simulink model "Template"  (Simulink 7.3)
settings: Solver=ode45  StartTime=0.0  StopTime=10.0  RelTol=1e-3
undefined symbols (not defined in the file): eta1_0_real, v1_0_real, velocitySatValues1
libraries: dspmtrx3 x21, simulink x14, dspindex x5, marine_gnc x4, simulink_extras x1, dspinverses x1
(part 1 of 4)
settings Model: Creator=mcl  LastModifiedBy=mcl

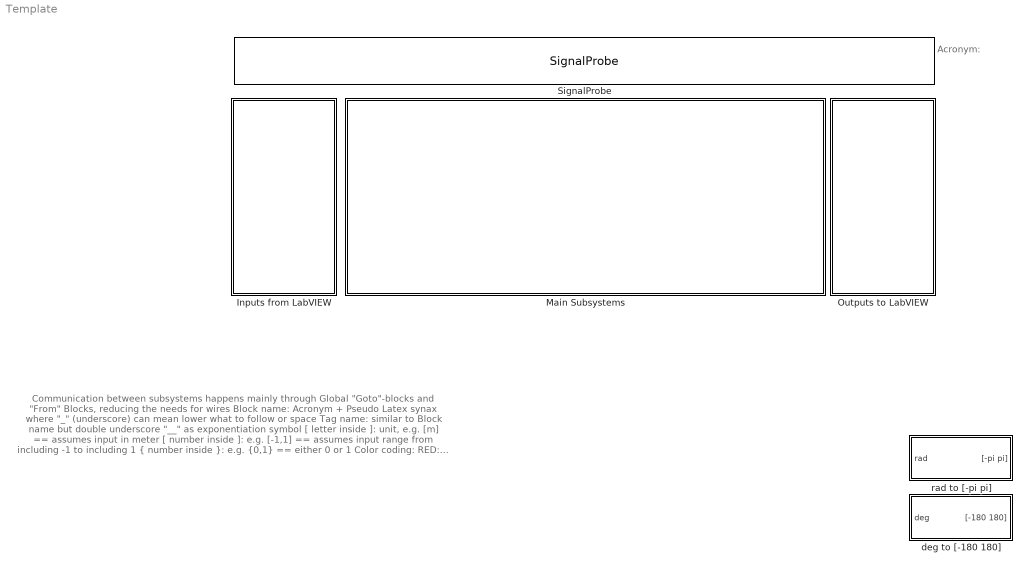
== system Template ==
  note: Communication between subsystems happens mainly through Global "Goto"-blocks and "From" Blocks,
      | reducing the needs for wires
      |
      | Block name: Acronym + Pseudo Latex synax where "_" (underscore) can mean lower what to follow or space
      | Tag name: similar to Block name but double underscore "__" as exponentiation symbol
      |
      | [ letter inside ]: unit, e.g. [m] == assumes input in meter
      | [ number inside ]: e.g. [-1,1] == assumes input range from including -1 to including 1
      | { number inside }:  e.g. {0,1} == either 0 or 1
      |
      | Color coding:
      | RED: Sinks (output ports, terminators, to workspace blocks, etc.)
      | GREEN Sources (inputs ports, constants, etc.)
      | CYAN: Memory blocks: Integrators, unit delays, memory, transfer functions, state space blocks, etc
      | GRAY: Logics blocks: Logic action ports, subsystem enable, etc.
      | ORANGE: GOTO blocks
      | MAGENTA: FROM blocks
      | YELLOW: All remaining blocks,
  note: Acronym:
  Inputs from LabVIEW : Subsystem
  Main Subsystems : Subsystem
  Outputs to LabVIEW : Subsystem
  SignalProbe : S-Function  Description=Use this block with SIT.  FunctionName=SignalProbe  Parameters=1  EnableBusSupport=off
      settings: PreSaveFcn=NISIT_ModelVars;
      mask Description: The LabVIEW Simulation Interface Toolkit uses the SignalProbe block to probe the signals in the model. The SignalProbe block must be on the top level of the model hierarchy. You can have only one SignalProbe block per model file. Do not rename the SignalProbe block. Do not change the name of another model block to SignalProbe.
  deg to [-180 180] : Subsystem
      mask Type: deg to -180/180
      mask Description: Converts an angle in deg to between -180 and 180
      mask Display: disp('[0 360] to [-180 180]')
  rad to [-pi pi] : Subsystem
      mask Type: rad to pi/pi
      mask Description: Converts an angle in rad to between -pi and pi
      mask Display: disp('[0 2pi] to [-pi pi]')

== system Template/Inputs from LabVIEW ==
  Control Input Selector : Constant  Value=0
  Control Mode Selector : Constant  Value=0
  Dynamic Positioning : Subsystem
  Enable CSE1 : Constant  Value=0
  LOS LgV backstepping II : Subsystem
  Linear Simulator : Subsystem
  Path : Subsystem
  PlayStation3 : Subsystem
  tag scope: Control_Input_Selector=global, Control_Mode_Selector=global, Enable_CSE1=global
  wires:
  Control Mode Selector/1 -> [Control_Mode_Selector]
  Control Input Selector/1 -> [Control_Input_Selector]
  Enable CSE1/1 -> [Enable_CSE1]

== system Template/Main Subsystems ==
  C/S Enterprise 1 : Subsystem
  Control : Subsystem
  Guidance : Subsystem
  Naviagation : Subsystem
  Plant : Subsystem

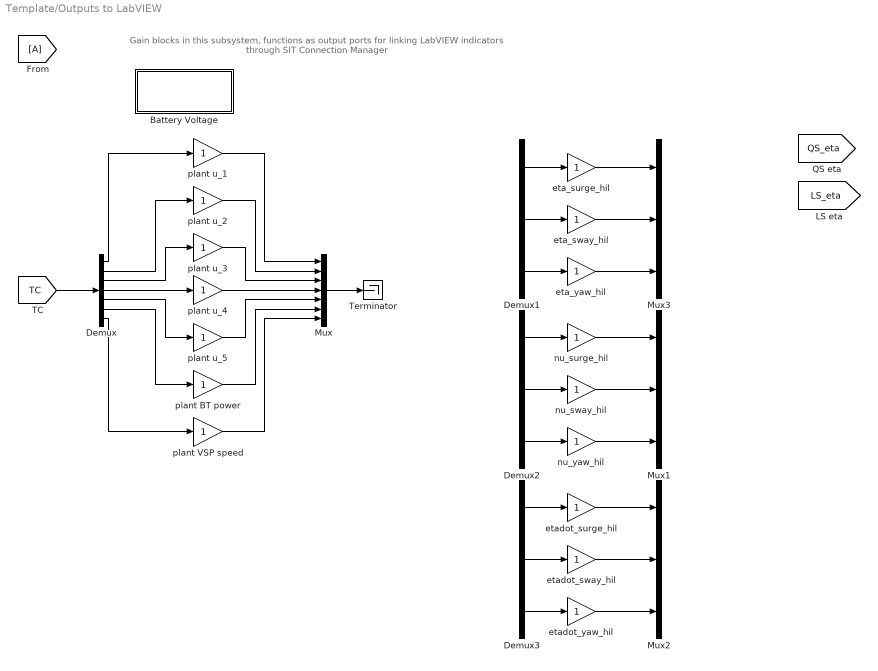
== system Template/Outputs to LabVIEW ==
  note: Gain blocks in this subsystem, functions as output ports for linking LabVIEW indicators through SIT Connection Manager
  Battery Voltage : Subsystem
  Demux : Demux  Outputs=7
  Demux1 : Demux  Outputs=3
  Demux2 : Demux  Outputs=3
  Demux3 : Demux  Outputs=3
  Mux : Mux  Inputs=7
  Mux1 : Mux  Inputs=3
  Mux2 : Mux  Inputs=3
  Mux3 : Mux  Inputs=3
  Terminator : Terminator
  eta_surge_hil : Gain  ParameterDataType=fixdt(1, 16)  ParameterScaling=2^0  OutDataType=fixdt(1, 16)  OutScaling=2^0
  eta_sway_hil : Gain  ParameterDataType=fixdt(1, 16)  ParameterScaling=2^0  OutDataType=fixdt(1, 16)  OutScaling=2^0
  eta_yaw_hil : Gain  ParameterDataType=fixdt(1, 16)  ParameterScaling=2^0  OutDataType=fixdt(1, 16)  OutScaling=2^0
  etadot_surge_hil : Gain  ParameterDataType=fixdt(1, 16)  ParameterScaling=2^0  OutDataType=fixdt(1, 16)  OutScaling=2^0
  etadot_sway_hil : Gain  ParameterDataType=fixdt(1, 16)  ParameterScaling=2^0  OutDataType=fixdt(1, 16)  OutScaling=2^0
  etadot_yaw_hil : Gain  ParameterDataType=fixdt(1, 16)  ParameterScaling=2^0  OutDataType=fixdt(1, 16)  OutScaling=2^0
  nu_surge_hil : Gain  ParameterDataType=fixdt(1, 16)  ParameterScaling=2^0  OutDataType=fixdt(1, 16)  OutScaling=2^0
  nu_sway_hil : Gain  ParameterDataType=fixdt(1, 16)  ParameterScaling=2^0  OutDataType=fixdt(1, 16)  OutScaling=2^0
  nu_yaw_hil : Gain  ParameterDataType=fixdt(1, 16)  ParameterScaling=2^0  OutDataType=fixdt(1, 16)  OutScaling=2^0
  plant BT power : Gain  ParameterDataType=fixdt(1, 16)  ParameterScaling=2^0  OutDataType=fixdt(1, 16)  OutScaling=2^0
  plant VSP speed : Gain  ParameterDataType=fixdt(1, 16)  ParameterScaling=2^0  OutDataType=fixdt(1, 16)  OutScaling=2^0
  plant u_{1..5} (5 alike) : Gain  ParameterDataType=fixdt(1, 16)  ParameterScaling=2^0  OutDataType=fixdt(1, 16)  OutScaling=2^0
  wires:
  Demux/1 -> plant u_1/1
  Demux/2 -> plant u_2/1
  Demux/3 -> plant u_3/1
  Demux/4 -> plant u_4/1
  plant u_4/1 -> Mux/4
  plant u_1/1 -> Mux/1
  plant u_2/1 -> Mux/2
  plant u_3/1 -> Mux/3
  Demux/5 -> plant u_5/1
  Demux/6 -> plant BT power/1
  Demux/7 -> plant VSP speed/1
  plant u_5/1 -> Mux/5
  plant BT power/1 -> Mux/6
  plant VSP speed/1 -> Mux/7
  nu_yaw_hil/1 -> Mux1/3
  nu_sway_hil/1 -> Mux1/2
  nu_surge_hil/1 -> Mux1/1
  Demux2/3 -> nu_yaw_hil/1
  Demux2/2 -> nu_sway_hil/1
  Demux2/1 -> nu_surge_hil/1
  eta_sway_hil/1 -> Mux3/2
  eta_yaw_hil/1 -> Mux3/3
  eta_surge_hil/1 -> Mux3/1
  Demux1/3 -> eta_yaw_hil/1
  Demux1/2 -> eta_sway_hil/1
  Demux1/1 -> eta_surge_hil/1
  etadot_sway_hil/1 -> Mux2/2
  etadot_yaw_hil/1 -> Mux2/3
  etadot_surge_hil/1 -> Mux2/1
  Demux3/3 -> etadot_yaw_hil/1
  Demux3/2 -> etadot_sway_hil/1
  Demux3/1 -> etadot_surge_hil/1
  [TC] -> Demux/1
  Mux/1 -> Terminator/1

== system Template/deg to [-180 180] ==
  deg : Inport  OutDataType=sfix(16)  OutScaling=2^0
  Constant : Constant  Value=2*180  OutDataType=sfix(16)  OutScaling=2^0
  Gain : Gain  Gain=180  ParameterDataType=sfix(16)  ParameterScaling=2^0  OutDataType=sfix(16)  OutScaling=2^0  SaturateOnIntegerOverflow=on  OutDataTypeStr=Inherit: Same as input  ParamDataTypeStr=Inherit: Same as input
  Math Function : Math  Operator=rem  OutDataType=sfix(16)  OutScaling=2^0  SaturateOnIntegerOverflow=on
  Saturation : Saturate  UpperLimit=1e10  LowerLimit=-1e10
  Sign : Signum
  Sum : Sum  Inputs=|+-  OutDataType=sfix(16)  OutScaling=2^0  SaturateOnIntegerOverflow=on
  Sum1 : Sum  Inputs=|++  OutDataType=sfix(16)  OutScaling=2^0  SaturateOnIntegerOverflow=on
  "[-180 180]" : Outport  OutDataType=sfix(16)  OutScaling=2^0
  wires:
  Sum/1 -> "[-180 180]"/1
  Math Function/1 -> Sum/1
  Constant/1 -> Math Function/2
  Sum1/1 -> Math Function/1
  Gain/1 -> Sum1/2, Sum/2
  Sign/1 -> Gain/1
  deg/1 -> Saturation/1
  Saturation/1 -> Sign/1, Sum1/1

== system Template/rad to [-pi pi] ==
  rad : Inport  OutDataType=sfix(16)  OutScaling=2^0
  Constant : Constant  Value=2*pi  OutDataType=sfix(16)  OutScaling=2^0
  Gain : Gain  Gain=pi  ParameterDataType=sfix(16)  ParameterScaling=2^0  OutDataType=sfix(16)  OutScaling=2^0  SaturateOnIntegerOverflow=on  OutDataTypeStr=Inherit: Same as input  ParamDataTypeStr=Inherit: Same as input
  Math Function : Math  Operator=rem  OutDataType=sfix(16)  OutScaling=2^0  SaturateOnIntegerOverflow=on
  Saturation : Saturate  UpperLimit=1e10  LowerLimit=-1e10
  Sign : Signum
  Sum : Sum  Inputs=|+-  OutDataType=sfix(16)  OutScaling=2^0  SaturateOnIntegerOverflow=on
  Sum1 : Sum  Inputs=|++  OutDataType=sfix(16)  OutScaling=2^0  SaturateOnIntegerOverflow=on
  "[-pi pi]" : Outport  OutDataType=sfix(16)  OutScaling=2^0
  wires:
  Saturation/1 -> Sum1/1, Sign/1
  rad/1 -> Saturation/1
  Sign/1 -> Gain/1
  Gain/1 -> Sum/2, Sum1/2
  Sum1/1 -> Math Function/1
  Constant/1 -> Math Function/2
  Math Function/1 -> Sum/1
  Sum/1 -> "[-pi pi]"/1

== system Template/Inputs from LabVIEW/Dynamic Positioning ==
  K_d : Subsystem
  K_d_Surge : Constant  Value=50
  K_d_Sway : Constant  Value=30
  K_d_Yaw : Constant  Value=5
  K_i : Subsystem
  K_i_Surge : Constant  Value=0
  K_i_Sway : Constant  Value=0
  K_i_Yaw : Constant  Value=0
  K_p : Subsystem
  K_p_Surge : Constant  Value=2*1.5*2
  K_p_Sway : Constant  Value=2*10*2
  K_p_Yaw : Constant  Value=0.5*3
  Reset integrator : Constant  Value=0
  Setpoint : Subsystem
  tag scope: DP_Reset_integrator=global
  wires:
  Reset integrator/1 -> [DP_Reset_integrator]
  K_p_Surge/1 -> K_p/1(11)
  K_p_Sway/1 -> K_p/2(22)
  K_p_Yaw/1 -> K_p/3(33)
  K_d_Surge/1 -> K_d/1(11)
  K_d_Sway/1 -> K_d/2(22)
  K_d_Yaw/1 -> K_d/3(33)
  K_i_Surge/1 -> K_i/1(11)
  K_i_Sway/1 -> K_i/2(22)
  K_i_Yaw/1 -> K_i/3(33)

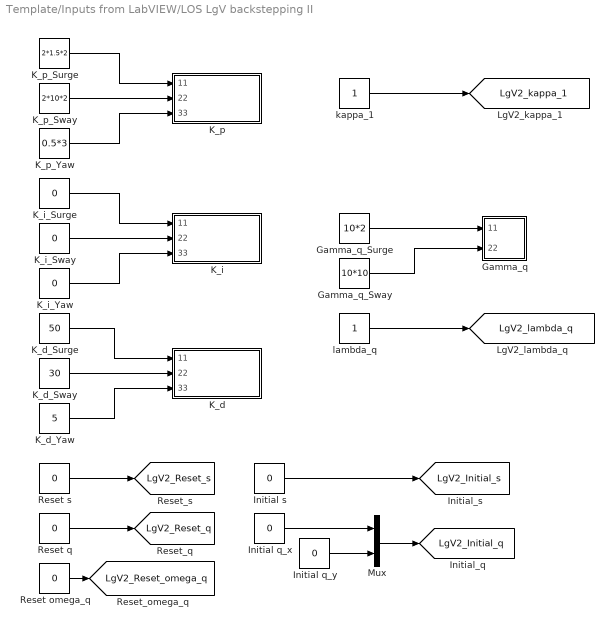
== system Template/Inputs from LabVIEW/LOS LgV backstepping II ==
  Gamma_q : Subsystem
  Gamma_q_Surge : Constant  Value=10*2
  Gamma_q_Sway : Constant  Value=10*10
  Initial q_x : Constant  Value=0  OutDataType=fixdt(1, 16)  OutScaling=2^0
  Initial q_y : Constant  Value=0  OutDataType=fixdt(1, 16)  OutScaling=2^0
  Initial s : Constant  Value=0  OutDataType=fixdt(1, 16)  OutScaling=2^0
  K_d : Subsystem
  K_d_Surge : Constant  Value=50
  K_d_Sway : Constant  Value=30
  K_d_Yaw : Constant  Value=5
  K_i : Subsystem
  K_i_Surge : Constant  Value=0
  K_i_Sway : Constant  Value=0
  K_i_Yaw : Constant  Value=0
  K_p : Subsystem
  K_p_Surge : Constant  Value=2*1.5*2
  K_p_Sway : Constant  Value=2*10*2
  K_p_Yaw : Constant  Value=0.5*3
  Mux : Mux  Inputs=2
  Reset omega_q : Constant  Value=0
  Reset q : Constant  Value=0
  Reset s : Constant  Value=0
  kappa_1 : Constant
  lambda_q : Constant
  tag scope: LgV2_Initial_q=global, LgV2_Initial_s=global, LgV2_Reset_omega_q=global, LgV2_Reset_q=global, LgV2_Reset_s=global, LgV2_kappa_1=global, LgV2_lambda_q=global
  wires:
  K_p_Surge/1 -> K_p/1(11)
  K_p_Sway/1 -> K_p/2(22)
  K_p_Yaw/1 -> K_p/3(33)
  K_d_Surge/1 -> K_d/1(11)
  K_d_Sway/1 -> K_d/2(22)
  K_d_Yaw/1 -> K_d/3(33)
  K_i_Surge/1 -> K_i/1(11)
  K_i_Sway/1 -> K_i/2(22)
  K_i_Yaw/1 -> K_i/3(33)
  Gamma_q_Surge/1 -> Gamma_q/1(11)
  Gamma_q_Sway/1 -> Gamma_q/2(22)
  kappa_1/1 -> [LgV2_kappa_1]
  lambda_q/1 -> [LgV2_lambda_q]
  Initial q_x/1 -> Mux/1
  Initial q_y/1 -> Mux/2
  Reset s/1 -> [LgV2_Reset_s]
  Reset q/1 -> [LgV2_Reset_q]
  Initial s/1 -> [LgV2_Initial_s]
  Mux/1 -> [LgV2_Initial_q]
  Reset omega_q/1 -> [LgV2_Reset_omega_q]

== system Template/Inputs from LabVIEW/Linear Simulator ==
  note: Enable Linear Simulator: Activation
      | Reset Linear Simulator integrator: Reset
      | Initial u: Initial speed in surge
      | Initial v: Initial speed in sway
      | Initial r: Initial speed in yaw
      | Initial x: Initial position in surge
      | Initial y: Initial position in sway
      | Initial psi: Initial heading
  Enable Linear Simulator : Constant  Value=0
  Initial psi [rad] : Constant  Value=0  OutDataType=fixdt(1, 16)  OutScaling=2^0
  Initial r [rad/s] : Constant  Value=0  OutDataType=fixdt(1, 16)  OutScaling=2^0
  Initial u [m/s] : Constant  Value=0  OutDataType=fixdt(1, 16)  OutScaling=2^0
  Initial v [m/s] : Constant  Value=0  OutDataType=fixdt(1, 16)  OutScaling=2^0
  Initial x [m] : Constant  Value=0  OutDataType=fixdt(1, 16)  OutScaling=2^0
  Initial y [m] : Constant  Value=0  OutDataType=fixdt(1, 16)  OutScaling=2^0
  Mux : Mux  Inputs=3
  Mux1 : Mux  Inputs=3
  Reset Linear Simulator integrator : Constant  Value=0
  tag scope: LS_Enable=global, LS_Initial_eta=global, LS_Initial_nu=global, LS_Reset=global
  wires:
  Enable Linear Simulator/1 -> [LS_Enable]
  Reset Linear Simulator integrator/1 -> [LS_Reset]
  Mux/1 -> [LS_Initial_nu]
  Initial r [rad/s]/1 -> Mux/3
  Initial v [m/s]/1 -> Mux/2
  Initial u [m/s]/1 -> Mux/1
  Mux1/1 -> [LS_Initial_eta]
  Initial psi [rad]/1 -> Mux1/3
  Initial y [m]/1 -> Mux1/2
  Initial x [m]/1 -> Mux1/1

== system Template/Inputs from LabVIEW/Path ==
  note: u_d: Desired surge speed of vessel
      | Path Selector: Workaround parameter for switching between linear path(==0) and ellipse path(==1)
      | x_dmax: Upper limit of desired x-ooordinate
      | x_dmin: Lower limit of desired x-coordiante
      | y_dmax: Upper limit of desired y-ooordinate
      | y_dmin: Lower limit of desired y-coordiante
      | Delta: Lookahead distance for LOS guidance
      | my: Gradient path minimizing tuning value
  Delta [m] : Constant  Value=2  OutDataType=fixdt(1, 16)  OutScaling=2^0
  Ellipse : Subsystem
  Linear : Subsystem
  Path Selector  [-] : Constant  Value=0
  my [-] : Constant  Value=10  OutDataType=fixdt(1, 16)  OutScaling=2^0
  u_d [m] : Constant  Value=0.15  OutDataType=fixdt(1, 16)  OutScaling=2^0
  x_dmax [m] : Constant  Value=40
  x_dmin [m] : Constant  Value=-40
  y_dmax [m] : Constant  Value=7
  y_dmin [m] : Constant  Value=-7
  tag scope: Delta=global, Path_Selector=global, my=global, u_d=global, x_dmax=global, x_dmin=global, y_dmax=global, y_dmin=global
  wires:
  u_d [m]/1 -> [u_d]  "Desired speed [m/s]"
  Delta [m]/1 -> [Delta]  "Lookahead distance [m]"
  my [-]/1 -> [my]  "s tuning parameter"
  Path Selector  [-]/1 -> [Path_Selector]  "chosen path {0,1}"
  x_dmax [m]/1 -> [x_dmax]
  x_dmin [m]/1 -> [x_dmin]
  y_dmax [m]/1 -> [y_dmax]
  y_dmin [m]/1 -> [y_dmin]

== system Template/Inputs from LabVIEW/PlayStation3 ==
  note: Postive Y-axis of analog sticks points up (in the direction of the shoulder buttons)
      | Postive X-axis of analog sticks points to the right (in the direction of Triange, Circle, X and Square buttons)
      |
      | AS_LX: PS3 Analog Stick Left X-postition
      | AS_LY: PS3 Analog Stick Left Y-postition
      | AS_RX: PS3 Analog Stick Right X-postition
      | AS_RY: PS3 Analog Stick Right Y-postition
      | L2: PS3 bottom left sholderbutton
      | R2: PS3 bottom right shoulderbotton
      | PS3_BT_Power: PS3 command bow thruster power setpoint
      | PS3 _VSP_speed: PS3 command Voith Schneider Propeller speed
  "AS_LX [-] " : Constant  Value=0
  AS_LY [-] : Constant  Value=0
  AS_RX [-] : Constant  Value=0
  AS_RY [-] : Constant  Value=0
  L2 [-] : Constant  Value=0
  PS3_BT_Power  [-] : Constant  Value=0
  PS3_VSP_Speed  [-] : Constant  Value=0
  R2 [-] : Constant  Value=0
  ScalingLX : Gain  Gain=1/32767
  ScalingLY : Gain  Gain=1/32767
  ScalingRY : Gain  Gain=1/32767
  Scaling_RX : Gain  Gain=1/32767
  tag scope: PS3_AS_LX=global, PS3_AS_LY=global, PS3_AS_RX=global, PS3_AS_RY=global, PS3_BT_Power=global, PS3_L2=global, PS3_R2=global, PS3_VSP_Speed=global
  wires:
  PS3_VSP_Speed  [-]/1 -> [PS3_VSP_Speed]  "Voith Schnider Propeller Speed"
  PS3_BT_Power  [-]/1 -> [PS3_BT_Power]  "Bow Thruster Power"
  "AS_LX [-] "/1 -> ScalingLX/1  "x-position of left analog stick [-32767,32767]"
  ScalingLX/1 -> [PS3_AS_LX]  "x-position of left analog stick [-1,1]"
  AS_LY [-]/1 -> ScalingLY/1  "y-position of left analog stick [-32767,32767]"
  ScalingLY/1 -> [PS3_AS_LY]  "y-position of left analog stick [-1,1]"
  AS_RX [-]/1 -> Scaling_RX/1  "x-position of right analog stick  [-32767,32767]"
  Scaling_RX/1 -> [PS3_AS_RX]  "x-position of right analog stick  [-1,1]"
  ScalingRY/1 -> [PS3_AS_RY]  "y-position of right analog stick [-1,1]"
  AS_RY [-]/1 -> ScalingRY/1  "y-position of right analog stick [-32767,32767]"
  L2 [-]/1 -> [PS3_L2]  "L2 Button [-1,0]"
  R2 [-]/1 -> [PS3_R2]  "R2 Button [0,1]"

== system Template/Main Subsystems/C/S Enterprise 1 ==
  Linear dampning matrix : Subsystem
  Mass matrix : Subsystem
  Thruster configuration matrix : Subsystem
  tag scope: B=global, D_L=global, M=global
  wires:
  Mass matrix/1(M) -> [M]
  Linear dampning matrix/1(D_L) -> [D_L]
  Thruster configuration matrix/1(B) -> [B]

== system Template/Main Subsystems/Control ==
  Control Switch : Subsystem
  DP control : Subsystem
  LgV2 : Subsystem
  Thruster allocation : Subsystem

== system Template/Main Subsystems/Guidance ==
  Line-Of-Sight Path-Following : Subsystem

== system Template/Main Subsystems/Naviagation ==
  Input from SIT : Subsystem
  Navigation Switch : Subsystem

== system Template/Main Subsystems/Plant ==
  CSE1 : Subsystem
  Enable CSE1 : Constant  Value=0
  Enable Linear Simulator : Constant  Value=0
  Inverse : Product  Inputs=/  Multiplication=Matrix(*)
  Linear Simulator : Subsystem
      settings: MinAlgLoopOccurrences=on
  saturation : Subsystem
  tag scope: LS_eta=global, LS_etadot=global, LS_nu=global
  wires:
  Enable CSE1/1 -> CSE1/Enable
  Enable Linear Simulator/1 -> Linear Simulator/Enable
  saturation/1(sat_tau) -> Linear Simulator/1(tau)
  [tau] -> saturation/1(tau)
  [TC] -> CSE1/1(Thurster setting)
  Linear Simulator/1(eta_hil) -> [LS_eta]
  Linear Simulator/2(nu_hil) -> [LS_nu]
  Linear Simulator/3(etadot_hil) -> [LS_etadot]
  [M] -> Inverse/1
  Inverse/1 -> Linear Simulator/2(M_inv)
  [D_L] -> Linear Simulator/3(D_L)
  [LS_Reset] -> Linear Simulator/4(Reset)
  [LS_Initial_eta] -> Linear Simulator/5(eta_0)
  [LS_Initial_nu] -> Linear Simulator/6(nu_0)

== system Template/Outputs to LabVIEW/Battery Voltage ==
  note: Main battery is multipled by 2, since the voltage is halfed at measuring point
  Battery Bow Thruster : Gain  ParameterDataType=fixdt(1, 16)  ParameterScaling=2^0  OutDataType=fixdt(1, 16)  OutScaling=2^0
  Battery Main : Gain  Gain=2  ParameterDataType=fixdt(1, 16)  ParameterScaling=2^0  OutDataType=fixdt(1, 16)  OutScaling=2^0
  Battery Servo : Gain  ParameterDataType=fixdt(1, 16)  ParameterScaling=2^0  OutDataType=fixdt(1, 16)  OutScaling=2^0
  Terminator Bow Thruster Battery : Terminator
  Terminator Main Battery : Terminator
  Terminator Servo Battery : Terminator
  wires:
  [Battery_BT] -> Battery Bow Thruster/1
  Battery Bow Thruster/1 -> Terminator Bow Thruster Battery/1
  [Battery_Servo] -> Battery Servo/1
  Battery Servo/1 -> Terminator Servo Battery/1
  [Battery_Main] -> Battery Main/1
  Battery Main/1 -> Terminator Main Battery/1

== system Template/Inputs from LabVIEW/Dynamic Positioning/K_d ==
  note: Creating 3x3 diagonal matrix
  11 : Inport
  22 : Inport  Port=2
  33 : Inport  Port=3
  {12..13,21,23,31..32} (6 alike) : Constant  Value=0
  Mux : Mux  Inputs=9
  "[3x3]" : Reshape  OutputDimensionality=Customize  OutputDimensions=[3,3]
  tag scope: DP_K_d=global
  wires:
  "[3x3]"/1 -> [DP_K_d]
  33/1 -> Mux/9
  23/1 -> Mux/8
  13/1 -> Mux/7
  32/1 -> Mux/6
  22/1 -> Mux/5
  12/1 -> Mux/4
  31/1 -> Mux/3
  21/1 -> Mux/2
  11/1 -> Mux/1
  Mux/1 -> "[3x3]"/1

== system Template/Inputs from LabVIEW/Dynamic Positioning/K_i ==
  note: Creating 3x3 diagonal matrix
  11 : Inport
  22 : Inport  Port=2
  33 : Inport  Port=3
  {12..13,21,23,31..32} (6 alike) : Constant  Value=0
  Mux : Mux  Inputs=9
  "[3x3]" : Reshape  OutputDimensionality=Customize  OutputDimensions=[3,3]
  tag scope: DP_K_i=global
  wires:
  "[3x3]"/1 -> [DP_K_i]
  33/1 -> Mux/9
  23/1 -> Mux/8
  13/1 -> Mux/7
  32/1 -> Mux/6
  22/1 -> Mux/5
  12/1 -> Mux/4
  31/1 -> Mux/3
  21/1 -> Mux/2
  11/1 -> Mux/1
  Mux/1 -> "[3x3]"/1

== system Template/Inputs from LabVIEW/Dynamic Positioning/K_p ==
  note: Creating 3x3 diagonal matrix
  11 : Inport
  22 : Inport  Port=2
  33 : Inport  Port=3
  {12..13,21,23,31..32} (6 alike) : Constant  Value=0
  Mux : Mux  Inputs=9
  "[3x3]" : Reshape  OutputDimensionality=Customize  OutputDimensions=[3,3]
  tag scope: DP_K_p=global
  wires:
  Mux/1 -> "[3x3]"/1
  11/1 -> Mux/1
  21/1 -> Mux/2
  31/1 -> Mux/3
  12/1 -> Mux/4
  22/1 -> Mux/5
  32/1 -> Mux/6
  13/1 -> Mux/7
  23/1 -> Mux/8
  33/1 -> Mux/9
  "[3x3]"/1 -> [DP_K_p]

== system Template/Inputs from LabVIEW/Dynamic Positioning/Setpoint ==
  " y_d [m]" : Constant  Value=0
  Degrees to Radians : simulink_extras/Transformations/Degrees to Radians  SystemSampleTime=-1
  Mux : Mux  Inputs=3
  psi_d [deg] : Constant  Value=0
  x_d [m] : Constant  Value=0
  tag scope: Setpoint=global
  wires:
  Degrees to Radians/1 -> Mux/3
  psi_d [deg]/1 -> Degrees to Radians/1
  " y_d [m]"/1 -> Mux/2
  x_d [m]/1 -> Mux/1
  Mux/1 -> [Setpoint]

== system Template/Inputs from LabVIEW/LOS LgV backstepping II/Gamma_q ==
  11 : Inport
  22 : Inport  Port=2
  12 : Constant  Value=0
  21 : Constant  Value=0
  Mux : Mux
  "[2x2]" : Reshape  OutputDimensionality=Customize  OutputDimensions=[2,2]
  tag scope: LgV2_Gamma_q=global
  wires:
  Mux/1 -> "[2x2]"/1
  11/1 -> Mux/1
  21/1 -> Mux/2
  12/1 -> Mux/3
  22/1 -> Mux/4
  "[2x2]"/1 -> [LgV2_Gamma_q]

== system Template/Inputs from LabVIEW/LOS LgV backstepping II/K_d ==
  note: Creating 3x3 diagonal matrix
  11 : Inport
  22 : Inport  Port=2
  33 : Inport  Port=3
  {12..13,21,23,31..32} (6 alike) : Constant  Value=0
  Mux : Mux  Inputs=9
  "[3x3]" : Reshape  OutputDimensionality=Customize  OutputDimensions=[3,3]
  tag scope: LgV2_K_d=global
  wires:
  "[3x3]"/1 -> [LgV2_K_d]
  33/1 -> Mux/9
  23/1 -> Mux/8
  13/1 -> Mux/7
  32/1 -> Mux/6
  22/1 -> Mux/5
  12/1 -> Mux/4
  31/1 -> Mux/3
  21/1 -> Mux/2
  11/1 -> Mux/1
  Mux/1 -> "[3x3]"/1

== system Template/Inputs from LabVIEW/LOS LgV backstepping II/K_i ==
  note: Creating 3x3 diagonal matrix
  11 : Inport
  22 : Inport  Port=2
  33 : Inport  Port=3
  {12..13,21,23,31..32} (6 alike) : Constant  Value=0
  Mux : Mux  Inputs=9
  "[3x3]" : Reshape  OutputDimensionality=Customize  OutputDimensions=[3,3]
  tag scope: LgV2_K_i=global
  wires:
  "[3x3]"/1 -> [LgV2_K_i]
  33/1 -> Mux/9
  23/1 -> Mux/8
  13/1 -> Mux/7
  32/1 -> Mux/6
  22/1 -> Mux/5
  12/1 -> Mux/4
  31/1 -> Mux/3
  21/1 -> Mux/2
  11/1 -> Mux/1
  Mux/1 -> "[3x3]"/1

== system Template/Inputs from LabVIEW/LOS LgV backstepping II/K_p ==
  note: Creating 3x3 diagonal matrix
  11 : Inport
  22 : Inport  Port=2
  33 : Inport  Port=3
  {12..13,21,23,31..32} (6 alike) : Constant  Value=0
  Mux : Mux  Inputs=9
  "[3x3]" : Reshape  OutputDimensionality=Customize  OutputDimensions=[3,3]
  tag scope: LgV2_K_p=global
  wires:
  Mux/1 -> "[3x3]"/1
  11/1 -> Mux/1
  21/1 -> Mux/2
  31/1 -> Mux/3
  12/1 -> Mux/4
  22/1 -> Mux/5
  32/1 -> Mux/6
  13/1 -> Mux/7
  23/1 -> Mux/8
  33/1 -> Mux/9
  "[3x3]"/1 -> [LgV2_K_p]

== system Template/Inputs from LabVIEW/Path/Ellipse ==
  note: origin_x: ellipse origin x-coordinate
      | origin_y: ellipse origin y-coordinate
      | r_x: ellipse radius x-direction
      | r_y: ellipse radius y-direction
      | k: step scaling factor of path parameter
  k [-] : Constant  Value=pi/180*2  OutDataType=fixdt(1, 16)  OutScaling=2^0
  origin_x [m] : Constant  Value=4.5  OutDataType=fixdt(1, 16)  OutScaling=2^0
  origo_y [m] : Constant  Value=0  OutDataType=fixdt(1, 16)  OutScaling=2^0
  r_x [m] : Constant  Value=5.5  OutDataType=fixdt(1, 16)  OutScaling=2^0
  r_y [m] : Constant  Value=2  OutDataType=fixdt(1, 16)  OutScaling=2^0
  tag scope: k=global, origin_x=global, origin_y=global, r_x=global, r_y=global
  wires:
  origin_x [m]/1 -> [origin_x]  "x-coord. origin ellipse path [m]"
  origo_y [m]/1 -> [origin_y]  "y-coord. origin ellipse path [m]"
  r_x [m]/1 -> [r_x]  "radius ellipse path x-axis [m]"
  r_y [m]/1 -> [r_y]  "radius ellipse path y-axis [m]"
  k [-]/1 -> [k]  "step scaling factor ellipse path [-]"

== system Template/Inputs from LabVIEW/Path/Linear ==
  note: x_1: reference way-point x-coordinate
      | y_1: reference way-point y-coordinate
      | x_2: direction way-point x-coordinate
      | y_2: direction way-point y-coordinate
  x_1 [m] : Constant  Value=0  OutDataType=fixdt(1, 16)  OutScaling=2^0
  x_2 [m] : Constant  Value=5.5  OutDataType=fixdt(1, 16)  OutScaling=2^0
  y_1 [m] : Constant  Value=0  OutDataType=fixdt(1, 16)  OutScaling=2^0
  y_2 [m] : Constant  Value=2  OutDataType=fixdt(1, 16)  OutScaling=2^0
  tag scope: x_1=global, x_2=global, y_1=global, y_2=global
  wires:
  x_1 [m]/1 -> [x_1]  "x-coord. reference point path [m]"
  y_1 [m]/1 -> [y_1]  "y-coord, reference point path [m]"
  x_2 [m]/1 -> [x_2]  "x-coord, direction point path [m]"
  y_2 [m]/1 -> [y_2]  "y-coord, direction point path [m]"

== system Template/Main Subsystems/C/S Enterprise 1/Linear dampning matrix ==
  -N_r : Gain  Gain=-1  ParameterDataType=fixdt(1, 16)  ParameterScaling=2^0  OutDataType=fixdt(1, 16)  OutScaling=2^0
  -N_v : Gain  Gain=-1  ParameterDataType=fixdt(1, 16)  ParameterScaling=2^0  OutDataType=fixdt(1, 16)  OutScaling=2^0
  -X_u : Gain  Gain=-1  ParameterDataType=fixdt(1, 16)  ParameterScaling=2^0  OutDataType=fixdt(1, 16)  OutScaling=2^0
  -Y_v : Gain  Gain=-1  ParameterDataType=fixdt(1, 16)  ParameterScaling=2^0  OutDataType=fixdt(1, 16)  OutScaling=2^0
  -Y_vr : Gain  Gain=-1  ParameterDataType=fixdt(1, 16)  ParameterScaling=2^0  OutDataType=fixdt(1, 16)  OutScaling=2^0
  D_L_{12..13,21,31} (4 alike) : Constant  Value=0
  Linear Dampning matrix : Reshape  OutputDimensionality=Customize  OutputDimensions=[3,3]
  Mux : Mux  Inputs=9
  N_r : Constant  Value=-1.900
  N_v : Constant  Value=0.18140
  X_u : Constant  Value=-0.59739
  Y_r : Constant  Value=-7.250
  Y_v : Constant  Value=-3.50625
  D_L : Outport
  wires:
  -N_r/1 -> Mux/9
  -Y_vr/1 -> Mux/8
  D_L_13/1 -> Mux/7
  -N_v/1 -> Mux/6
  -Y_v/1 -> Mux/5
  D_L_12/1 -> Mux/4
  D_L_31/1 -> Mux/3
  D_L_21/1 -> Mux/2
  -X_u/1 -> Mux/1
  N_r/1 -> -N_r/1
  Y_r/1 -> -Y_vr/1
  N_v/1 -> -N_v/1
  Y_v/1 -> -Y_v/1
  Linear Dampning matrix/1 -> D_L/1
  Mux/1 -> Linear Dampning matrix/1
  X_u/1 -> -X_u/1

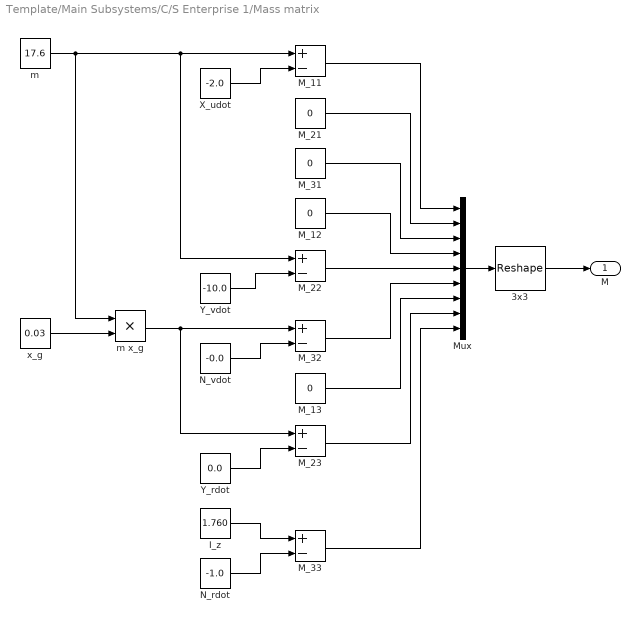
== system Template/Main Subsystems/C/S Enterprise 1/Mass matrix ==
  3x3 : Reshape  OutputDimensionality=Customize  OutputDimensions=[3,3]
  I_z : Constant  Value=1.760
  M_{11,22..23,32..33} (5 alike) : Sum  Inputs=+-
  M_{12..13,21,31} (4 alike) : Constant  Value=0
  Mux : Mux  Inputs=9
  N_rdot : Constant  Value=-1.0
  N_vdot : Constant  Value=-0.0
  X_udot : Constant  Value=-2.0
  Y_rdot : Constant  Value=0.0
  Y_vdot : Constant  Value=-10.0
  m : Constant  Value=17.6
  m x_g : Product  RndMeth=Zero
  x_g : Constant  Value=0.03
  M : Outport
  wires:
  3x3/1 -> M/1
  Mux/1 -> 3x3/1
  M_33/1 -> Mux/9
  M_23/1 -> Mux/8
  M_13/1 -> Mux/7
  M_32/1 -> Mux/6
  M_22/1 -> Mux/5
  M_12/1 -> Mux/4
  M_31/1 -> Mux/3
  M_21/1 -> Mux/2
  M_11/1 -> Mux/1
  N_rdot/1 -> M_33/2
  I_z/1 -> M_33/1
  Y_rdot/1 -> M_23/2
  N_vdot/1 -> M_32/2
  m x_g/1 -> M_23/1, M_32/1
  x_g/1 -> m x_g/2
  Y_vdot/1 -> M_22/2
  X_udot/1 -> M_11/2
  m/1 -> m x_g/1, M_22/1, M_11/1

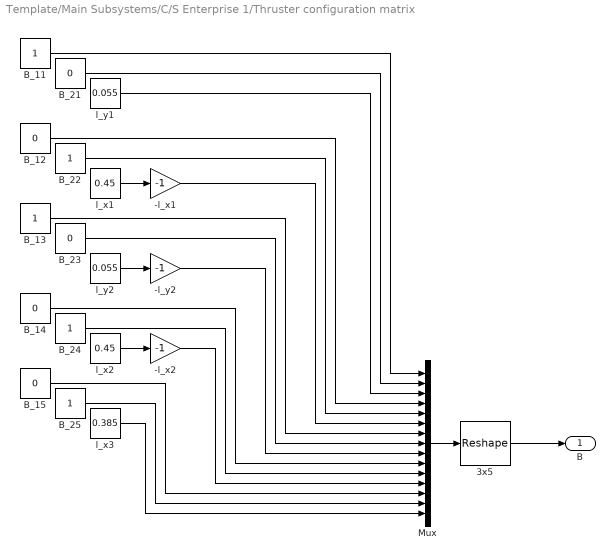
== system Template/Main Subsystems/C/S Enterprise 1/Thruster configuration matrix ==
  -l_x1 : Gain  Gain=-1
  -l_x2 : Gain  Gain=-1
  -l_y2 : Gain  Gain=-1
  3x5 : Reshape  OutputDimensionality=Customize  OutputDimensions=[3,5]
  B_{11,13,22,24..25} (5 alike) : Constant
  B_{12,14..15,21,23} (5 alike) : Constant  Value=0
  Mux : Mux  Inputs=15
  l_x1 : Constant  Value=0.45
  l_x2 : Constant  Value=0.45
  l_x3 : Constant  Value=0.385
  l_y1 : Constant  Value=0.055
  l_y2 : Constant  Value=0.055
  B : Outport
  wires:
  l_x3/1 -> Mux/15
  B_25/1 -> Mux/14
  B_15/1 -> Mux/13
  -l_x2/1 -> Mux/12
  -l_y2/1 -> Mux/9
  -l_x1/1 -> Mux/6
  l_x2/1 -> -l_x2/1
  B_24/1 -> Mux/11
  B_14/1 -> Mux/10
  l_y2/1 -> -l_y2/1
  B_23/1 -> Mux/8
  B_13/1 -> Mux/7
  l_x1/1 -> -l_x1/1
  B_22/1 -> Mux/5
  B_12/1 -> Mux/4
  l_y1/1 -> Mux/3
  B_21/1 -> Mux/2
  B_11/1 -> Mux/1
  3x5/1 -> B/1
  Mux/1 -> 3x5/1

== system Template/Main Subsystems/Control/Control Switch ==
  note: 0 - PS3 u input control
      | 1 - DP control
      | 2 - LgV2 control
  Control Mode : Constant  Value=0
  tau Switch : MultiPortSwitch  Inputs=2  zeroidx=on
  tag scope: tau=global
  wires:
  Control Mode/1 -> tau Switch/1
  [DP_tau] -> tau Switch/2
  [LgV2_tau] -> tau Switch/3
  tau Switch/1 -> [tau]

== system Template/Main Subsystems/Control/DP control ==
  note: Modified version of the DP control found in MSS toolbx
  Demux : Demux  Outputs=3
  Integrator : Integrator  ExternalReset=level
  Mux : Mux  Inputs=3
  Product : Product  Multiplication=Matrix(*)  OutDataType=fixdt(1, 16)  OutScaling=2^0  RndMeth=Zero
  Product1 : Product  Multiplication=Matrix(*)  OutDataType=fixdt(1, 16)  OutScaling=2^0  RndMeth=Zero
  Product2 : Product  Multiplication=Matrix(*)  OutDataType=fixdt(1, 16)  OutScaling=2^0  RndMeth=Zero
  Sum1 : Sum  Inputs=|+-  SaturateOnIntegerOverflow=on  InputSameDT=on  OutDataTypeStr=Inherit: Same as first input
  Sum2 : Sum  Inputs=+-|  SaturateOnIntegerOverflow=on  InputSameDT=on  OutDataTypeStr=Inherit: Same as first input
  Sum3 : Sum  Inputs=|++  SaturateOnIntegerOverflow=on  InputSameDT=on  OutDataTypeStr=Inherit: Same as first input
  Transposed rotation  matrix in yaw1 : marine_gnc/Models/ Kinematics/Transposed rotation  matrix in yaw  SystemSampleTime=-1
  "[-inf inf] to [-pi pi]" : marine_gnc/Utilities/Math Operations/[-inf inf] to [-pi pi]  SystemSampleTime=-1
  "[-inf inf] to [-pi pi]1" : marine_gnc/Utilities/Math Operations/[-inf inf] to [-pi pi]  SystemSampleTime=-1
  yaw angle : Fcn  Expr=u(3)
  tag scope: DP_tau=global
  wires:
  [DP_K_d] -> Product2/1
  [DP_K_i] -> Product1/1
  [DP_K_p] -> Product/1
  Product1/1 -> Sum3/2
  Product/1 -> Sum3/1
  Product2/1 -> Sum1/2
  "[-inf inf] to [-pi pi]"/1 -> Mux/3
  Demux/3 -> "[-inf inf] to [-pi pi]"/1
  "[-inf inf] to [-pi pi]1"/1 -> Transposed rotation  matrix in yaw1/1
  yaw angle/1 -> "[-inf inf] to [-pi pi]1"/1  "psi"
  [Reset_DP_integrator] -> Integrator/2
  [nu] -> Product2/2
  Sum2/1 -> Demux/1
  Transposed rotation  matrix in yaw1/1 -> Product/2, Integrator/1
  Sum3/1 -> Sum1/1
  Integrator/1 -> Product1/2
  [eta] -> Sum2/2, yaw angle/1
  Sum1/1 -> [DP_tau]
  [Setpoint] -> Sum2/1
  Demux/2 -> Mux/2
  Demux/1 -> Mux/1
  Mux/1 -> Transposed rotation  matrix in yaw1/2

== system Template/Main Subsystems/Control/LgV2 ==
  Auxilary functions g_q : Subsystem
  Auxiliary function g_s : Subsystem
  Control law : Subsystem
  R(psi) : Subsystem
  R^T : dspmtrx3/Transpose  SystemSampleTime=-1  Hermitian=off  overflowFlag=off
  Update laws : Subsystem
  V_1^q : Subsystem
  alpha : Subsystem
  alpha^q : Subsystem
  alpha^s : Subsystem
  psi : Selector  InputPortWidth=3  IndexOptions=Index vector (dialog)  Indices=[3]  OutputSizes=1
  sigma : Subsystem
  z_1 : Subsystem
  z_2 : Subsystem
  zeta : Subsystem
  tag scope: R_psi__T=global
  wires:
  psi/1 -> R(psi)/1(psi)
  [eta] -> psi/1
  R(psi)/1(R) -> R^T/1
  R^T/1 -> [R_psi__T]

== system Template/Main Subsystems/Control/Thruster allocation ==
  Saturation : Saturate  UpperLimit=1.0  LowerLimit=-1.0
  VSP030 BT040 : Subsystem
  tau to f_act : Subsystem
  tag scope: TC=global
  wires:
  [tau] -> tau to f_act/1(tau)
  tau to f_act/1(f_act) -> VSP030 BT040/1(f_act)
  VSP030 BT040/1(TC) -> Saturation/1
  Saturation/1 -> [TC]

== system Template/Main Subsystems/Guidance/Line-Of-Sight Path-Following ==
  Heading : Subsystem
  Line-Of-Sight : Subsystem
  Path : Subsystem
  Speed assigment : Subsystem

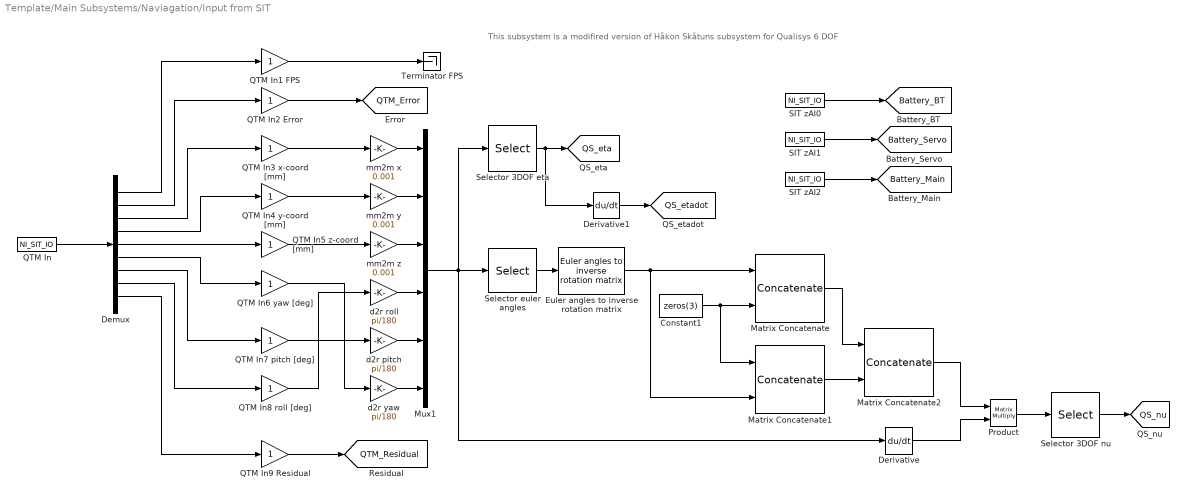
== system Template/Main Subsystems/Naviagation/Input from SIT ==
  note: This subsystem is a modifired version of Håkon Skåtuns subsystem for Qualisys 6 DOF
  Constant1 : Constant  Value=zeros(3)
  Demux : Demux  Outputs=9
  Derivative : Derivative
  Derivative1 : Derivative
  Euler angles to inverse rotation matrix : marine_gnc/Models/ Kinematics/Euler angles to inverse rotation matrix  SystemSampleTime=-1
  Matrix Concatenate : Concatenate  Mode=Multidimensional array
  Matrix Concatenate1 : Concatenate  Mode=Multidimensional array
  Matrix Concatenate2 : Concatenate  Mode=Multidimensional array  ConcatenateDimension=2
  Mux1 : Mux  Inputs=6
  Product : Product  Multiplication=Matrix(*)  RndMeth=Zero
  QTM In : S-Function  Priority=1  FunctionName=NI_SIT_IO  Parameters=width dtype portnum stime stype btype  EnableBusSupport=off  mask(SIT Inport){portnum=1, width=9, stime=-1, dtype=auto, stype=auto, btype=1}
      mask prompts: portnum "Port number:"; width "Port dimensions (-1 for dynamically sized):"; stime "Sample time (-1 for inherited):"; dtype "Data type:"; stype "Signal type:"; btype "Block type:"
      mask help: Use this inport on any level of nested subsystems to allow the LabVIEW Simulation Interface Toolkit to map hardware to it.
      mask init:
      | NI_SIT_IO_init;
      settings: CopyFcn=NI_SIT_IO_callbacks(1);  DeleteFcn=NI_SIT_IO_callbacks(2);
      mask StyleString: edit,edit,edit,popup(auto|double|single|int8|uint8|int16|uint16|int32|uint32|boolean),popup(auto|real|complex),edit
      mask CallbackString: NI_SIT_IO_callbacks(3);|||NI_SIT_IO_callbacks(4);||
      mask TabNameString: Parameters,Parameters,Parameters,Parameters,Parameters,Parameters
      mask Display:
      | patch([-x x], [-y y], [.90980 .81960 .32156]);
      | plot([0 -x x 0], [rad -y y rad]);
      | fprintf('SIT%d', portnum);
  QTM In1 FPS : Gain  ParameterDataType=fixdt(1, 16)  ParameterScaling=2^0  OutDataType=fixdt(1, 16)  OutScaling=2^0
  QTM In2 Error : Gain  ParameterDataType=fixdt(1, 16)  ParameterScaling=2^0  OutDataType=fixdt(1, 16)  OutScaling=2^0
  QTM In3 x-coord [mm] : Gain  ParameterDataType=fixdt(1, 16)  ParameterScaling=2^0  OutDataType=fixdt(1, 16)  OutScaling=2^0
  QTM In4 y-coord [mm] : Gain  ParameterDataType=fixdt(1, 16)  ParameterScaling=2^0  OutDataType=fixdt(1, 16)  OutScaling=2^0
  QTM In5 z-coord [mm] : Gain  ParameterDataType=fixdt(1, 16)  ParameterScaling=2^0  OutDataType=fixdt(1, 16)  OutScaling=2^0
  QTM In6 yaw [deg] : Gain  ParameterDataType=fixdt(1, 16)  ParameterScaling=2^0  OutDataType=fixdt(1, 16)  OutScaling=2^0
  QTM In7 pitch [deg] : Gain  ParameterDataType=fixdt(1, 16)  ParameterScaling=2^0  OutDataType=fixdt(1, 16)  OutScaling=2^0
  QTM In8 roll [deg] : Gain  ParameterDataType=fixdt(1, 16)  ParameterScaling=2^0  OutDataType=fixdt(1, 16)  OutScaling=2^0
  QTM In9 Residual : Gain  ParameterDataType=fixdt(1, 16)  ParameterScaling=2^0  OutDataType=fixdt(1, 16)  OutScaling=2^0
  SIT zAI0 : S-Function  Priority=2  FunctionName=NI_SIT_IO  Parameters=width dtype portnum stime stype btype  EnableBusSupport=off  mask(SIT Inport){portnum=2, width=-1, stime=-1, dtype=auto, stype=auto, btype=1}
      mask prompts: portnum "Port number:"; width "Port dimensions (-1 for dynamically sized):"; stime "Sample time (-1 for inherited):"; dtype "Data type:"; stype "Signal type:"; btype "Block type:"
      mask help: Use this inport on any level of nested subsystems to allow the LabVIEW Simulation Interface Toolkit to map hardware to it.
      mask init:
      | NI_SIT_IO_init;
      settings: CopyFcn=NI_SIT_IO_callbacks(1);  DeleteFcn=NI_SIT_IO_callbacks(2);
      mask StyleString: edit,edit,edit,popup(auto|double|single|int8|uint8|int16|uint16|int32|uint32|boolean),popup(auto|real|complex),edit
      mask CallbackString: NI_SIT_IO_callbacks(3);|||NI_SIT_IO_callbacks(4);||
      mask TabNameString: Parameters,Parameters,Parameters,Parameters,Parameters,Parameters
      mask Display:
      | patch([-x x], [-y y], [.90980 .81960 .32156]);
      | plot([0 -x x 0], [rad -y y rad]);
      | fprintf('SIT%d', portnum);
  SIT zAI1 : S-Function  Priority=3  FunctionName=NI_SIT_IO  Parameters=width dtype portnum stime stype btype  EnableBusSupport=off  mask(SIT Inport){portnum=3, width=-1, stime=-1, dtype=auto, stype=auto, btype=1}
      mask prompts: portnum "Port number:"; width "Port dimensions (-1 for dynamically sized):"; stime "Sample time (-1 for inherited):"; dtype "Data type:"; stype "Signal type:"; btype "Block type:"
      mask help: Use this inport on any level of nested subsystems to allow the LabVIEW Simulation Interface Toolkit to map hardware to it.
      mask init:
      | NI_SIT_IO_init;
      settings: CopyFcn=NI_SIT_IO_callbacks(1);  DeleteFcn=NI_SIT_IO_callbacks(2);
      mask StyleString: edit,edit,edit,popup(auto|double|single|int8|uint8|int16|uint16|int32|uint32|boolean),popup(auto|real|complex),edit
      mask CallbackString: NI_SIT_IO_callbacks(3);|||NI_SIT_IO_callbacks(4);||
      mask TabNameString: Parameters,Parameters,Parameters,Parameters,Parameters,Parameters
      mask Display:
      | patch([-x x], [-y y], [.90980 .81960 .32156]);
      | plot([0 -x x 0], [rad -y y rad]);
      | fprintf('SIT%d', portnum);
  SIT zAI2 : S-Function  Priority=4  FunctionName=NI_SIT_IO  Parameters=width dtype portnum stime stype btype  EnableBusSupport=off  mask(SIT Inport){portnum=4, width=-1, stime=-1, dtype=auto, stype=auto, btype=1}
      mask prompts: portnum "Port number:"; width "Port dimensions (-1 for dynamically sized):"; stime "Sample time (-1 for inherited):"; dtype "Data type:"; stype "Signal type:"; btype "Block type:"
      mask help: Use this inport on any level of nested subsystems to allow the LabVIEW Simulation Interface Toolkit to map hardware to it.
      mask init:
      | NI_SIT_IO_init;
      settings: CopyFcn=NI_SIT_IO_callbacks(1);  DeleteFcn=NI_SIT_IO_callbacks(2);
      mask StyleString: edit,edit,edit,popup(auto|double|single|int8|uint8|int16|uint16|int32|uint32|boolean),popup(auto|real|complex),edit
      mask CallbackString: NI_SIT_IO_callbacks(3);|||NI_SIT_IO_callbacks(4);||
      mask TabNameString: Parameters,Parameters,Parameters,Parameters,Parameters,Parameters
      mask Display:
      | patch([-x x], [-y y], [.90980 .81960 .32156]);
      | plot([0 -x x 0], [rad -y y rad]);
      | fprintf('SIT%d', portnum);
  Selector 3DOF eta : Selector  InputPortWidth=6  IndexOptions=Index vector (dialog)  Indices=[1 2 6]  OutputSizes=1
  Selector 3DOF nu : Selector  InputPortWidth=6  IndexOptions=Index vector (dialog)  Indices=[1 2 6]  OutputSizes=1
  Selector euler angles : Selector  InputPortWidth=6  IndexOptions=Index vector (dialog)  Indices=[4 5 6]  OutputSizes=1
  Terminator FPS : Terminator
  d2r pitch : Gain  Gain=pi/180  ParameterDataType=fixdt(1, 16)  ParameterScaling=2^0  OutDataType=fixdt(1, 16)  OutScaling=2^0
  d2r roll : Gain  Gain=pi/180  ParameterDataType=fixdt(1, 16)  ParameterScaling=2^0  OutDataType=fixdt(1, 16)  OutScaling=2^0
  d2r yaw : Gain  Gain=pi/180  ParameterDataType=fixdt(1, 16)  ParameterScaling=2^0  OutDataType=fixdt(1, 16)  OutScaling=2^0
  mm2m x : Gain  Gain=0.001
  mm2m y : Gain  Gain=0.001
  mm2m z : Gain  Gain=0.001
  tag scope: Battery_BT=global, Battery_Main=global, Battery_Servo=global, QS_eta=global, QS_etadot=global, QS_nu=global, QTM_Error=global, QTM_Residual=global
  wires:
  SIT zAI2/1 -> [Battery_Main]
  SIT zAI1/1 -> [Battery_Servo]
  SIT zAI0/1 -> [Battery_BT]
  Derivative1/1 -> [QS_etadot]
  QTM In8 roll [deg]/1 -> d2r roll/1
  QTM In6 yaw [deg]/1 -> d2r yaw/1
  QTM In7 pitch [deg]/1 -> d2r pitch/1
  QTM In5 z-coord [mm]/1 -> mm2m z/1
  QTM In4 y-coord [mm]/1 -> mm2m y/1
  QTM In3 x-coord [mm]/1 -> mm2m x/1
  Demux/9 -> QTM In9 Residual/1
  Demux/8 -> QTM In8 roll [deg]/1
  Demux/7 -> QTM In7 pitch [deg]/1
  Demux/6 -> QTM In6 yaw [deg]/1
  Demux/5 -> QTM In5 z-coord [mm]/1
  Demux/4 -> QTM In4 y-coord [mm]/1
  Demux/3 -> QTM In3 x-coord [mm]/1
  Demux/2 -> QTM In2 Error/1
  Demux/1 -> QTM In1 FPS/1
  QTM In/1 -> Demux/1
  QTM In9 Residual/1 -> [QTM_Residual]
  QTM In2 Error/1 -> [QTM_Error]
  QTM In1 FPS/1 -> Terminator FPS/1
  Selector 3DOF nu/1 -> [QS_nu]
  Product/1 -> Selector 3DOF nu/1
  Selector euler angles/1 -> Euler angles to inverse rotation matrix/1
  d2r roll/1 -> Mux1/4
  d2r pitch/1 -> Mux1/5
  d2r yaw/1 -> Mux1/6
  mm2m x/1 -> Mux1/1
  mm2m y/1 -> Mux1/2
  mm2m z/1 -> Mux1/3
  Constant1/1 -> Matrix Concatenate1/1, Matrix Concatenate/2
  Derivative/1 -> Product/2
  Matrix Concatenate2/1 -> Product/1
  Matrix Concatenate1/1 -> Matrix Concatenate2/2
  Matrix Concatenate/1 -> Matrix Concatenate2/1
  Euler angles to inverse rotation matrix/1 -> Matrix Concatenate1/2, Matrix Concatenate/1
  Selector 3DOF eta/1 -> [QS_eta], Derivative1/1
  Mux1/1 -> Selector 3DOF eta/1, Derivative/1, Selector euler angles/1

== system Template/Main Subsystems/Naviagation/Navigation Switch ==
  Controller Input Selector : Constant  Value=0
  eta Switch : MultiPortSwitch  Inputs=2  zeroidx=on
  etadot Switch : MultiPortSwitch  Inputs=2  zeroidx=on
  nu Switch : MultiPortSwitch  Inputs=2  zeroidx=on
  tag scope: eta=global, etadot=global, nu=global
  wires:
  Controller Input Selector/1 -> eta Switch/1, nu Switch/1, etadot Switch/1
  [QS_eta] -> eta Switch/2
  [LS_eta] -> eta Switch/3
  [QS_nu] -> nu Switch/2
  [LS_nu] -> nu Switch/3
  [QS_etadot] -> etadot Switch/2
  [LS_etadot] -> etadot Switch/3
  eta Switch/1 -> [eta]
  nu Switch/1 -> [nu]
  etadot Switch/1 -> [etadot]

== system Template/Main Subsystems/Plant/CSE1 ==
  note: This subsystem is a modifired version of Håkon Skåtuns subsystem CSE1
  Thurster setting : Inport
  Enable : EnablePort  StatesWhenEnabling=reset
  Bow Thruster : Subsystem
  Demux : Demux  Outputs=7
  "Voith Schneider Propeller " : Subsystem
  wires:
  Thurster setting/1 -> Demux/1
  Demux/1 -> "Voith Schneider Propeller "/1(Port VSP y u_1)
  Demux/2 -> "Voith Schneider Propeller "/2(Port VSP x u_2)
  Demux/3 -> "Voith Schneider Propeller "/3(Starboard VSP y u_3)
  Demux/4 -> "Voith Schneider Propeller "/4(Starboard VSP x u_4)
  Demux/7 -> "Voith Schneider Propeller "/5(VSP Speed)
  Demux/5 -> Bow Thruster/1(Bow Thruster Direction u_5)
  Demux/6 -> Bow Thruster/2(Bow Thruster Power)

== system Template/Main Subsystems/Plant/Linear Simulator ==
  tau : Inport
  M_inv : Inport  Port=2
  D_L : Inport  Port=3
  Reset : Inport  Port=4
  eta_0 : Inport  Port=5
  nu_0 : Inport  Port=6
  Enable : EnablePort  StatesWhenEnabling=reset
  Linear Vessel Dynamics : Subsystem
  eta_hil : Outport
  nu_hil : Outport  Port=2
  etadot_hil : Outport  Port=3
  wires:
  tau/1 -> Linear Vessel Dynamics/1(tau)
  Linear Vessel Dynamics/1(eta) -> eta_hil/1
  Linear Vessel Dynamics/2(nu) -> nu_hil/1
  Linear Vessel Dynamics/3(etadot) -> etadot_hil/1
  M_inv/1 -> Linear Vessel Dynamics/2(M_inv)
  D_L/1 -> Linear Vessel Dynamics/3(D_L)
  Reset/1 -> Linear Vessel Dynamics/4(Reset)
  eta_0/1 -> Linear Vessel Dynamics/5(eta_0)
  nu_0/1 -> Linear Vessel Dynamics/6(nu_0)

== system Template/Main Subsystems/Plant/saturation ==
  tau : Inport  OutDataType=sfix(16)  OutScaling=2^0
  Demux : Demux  Outputs=3
  Mux1 : Mux  Inputs=3
  Saturation : Saturate  UpperLimit=3  LowerLimit=-2.6  OutDataType=fixdt(1, 16)  OutScaling=2^0
  Saturation1 : Saturate  UpperLimit=3  LowerLimit=-3.5  OutDataType=fixdt(1, 16)  OutScaling=2^0
  Saturation2 : Saturate  UpperLimit=1.6  LowerLimit=-1.5  OutDataType=fixdt(1, 16)  OutScaling=2^0
  plant tau_surge : Gain  ParameterDataType=fixdt(1, 16)  ParameterScaling=2^0  OutDataType=fixdt(1, 16)  OutScaling=2^0
  plant tau_sway : Gain  ParameterDataType=fixdt(1, 16)  ParameterScaling=2^0  OutDataType=fixdt(1, 16)  OutScaling=2^0
  plant tau_yaw : Gain  ParameterDataType=fixdt(1, 16)  ParameterScaling=2^0  OutDataType=fixdt(1, 16)  OutScaling=2^0
  sat_tau : Outport  OutDataType=sfix(16)  OutScaling=2^0
  wires:
  Mux1/1 -> sat_tau/1
  tau/1 -> Demux/1
  Saturation/1 -> plant tau_surge/1
  Demux/1 -> Saturation/1
  Demux/2 -> Saturation1/1
  Saturation1/1 -> plant tau_sway/1
  plant tau_surge/1 -> Mux1/1
  plant tau_sway/1 -> Mux1/2
  Demux/3 -> Saturation2/1
  Saturation2/1 -> plant tau_yaw/1
  plant tau_yaw/1 -> Mux1/3

== system Template/Main Subsystems/Control/LgV2/Auxilary functions g_q ==
  g_q eq : Subsystem
  g_q^q eq : Subsystem
  g_q^s eq : Subsystem
  g_q^t eq : Subsystem
  tag scope: g_q=global, g_q__q=global, g_q__s=global, g_q__t=global
  wires:
  g_q eq/1(g_q) -> [g_q]
  [psi_los__q] -> g_q eq/2(psi_los^q), g_q^q eq/2(psi_los^q), g_q^s eq/2(psi_los^q), g_q^t eq/1(psi_los^q)
  [f_q] -> g_q eq/1(f_q), g_q^q eq/1(f_q), g_q^s eq/1(f_q)
  [f_q__q] -> g_q^q eq/3(f_q^q)
  [psi_los__q__2] -> g_q^q eq/4(psi_los^q^2)
  g_q^q eq/1(g_q^q) -> [g_q__q]
  g_q^s eq/1(g_q^s) -> [g_q__s]
  [f_q__s] -> g_q^s eq/3(f_q^s)
  [psi_los__qs] -> g_q^s eq/4(psi_los^qs)
  g_q^t eq/1(g_q^t) -> [g_q__t]
  [f_q__t] -> g_q^t eq/2(f_q^t)

== system Template/Main Subsystems/Control/LgV2/Auxiliary function g_s ==
  g_s eq : Subsystem
  g_s^q eq : Subsystem
  g_s^s eq : Subsystem
  g_s^t eq : Subsystem
  tag scope: g_s=global, g_s__q=global, g_s__s=global, g_s__t=global
  wires:
  [f_s] -> g_s eq/1(f_s), g_s^q eq/1(f_s), g_s^s eq/1(f_s)
  [psi_los__s] -> g_s eq/2(psi_los^s), g_s^q eq/2(psi_los^s), g_s^s eq/2(psi_los^s), g_s^t eq/1(psi_los^s)
  g_s eq/1(g_s) -> [g_s]
  [f_s__q] -> g_s^q eq/3(f_s^q)
  [psi_los__qs] -> g_s^q eq/4(psi_los^sq)
  g_s^q eq/1(g_s^q) -> [g_s__q]
  g_s^s eq/1(g_s^s) -> [g_s__s]
  [f_s__s] -> g_s^s eq/3(f_s^s)
  [psi_los__s__2] -> g_s^s eq/4(psi_los^s^2)
  g_s^t eq/1(g_a^t) -> [g_s__t]
  [f_s__t] -> g_s^t eq/2(f_s^t)

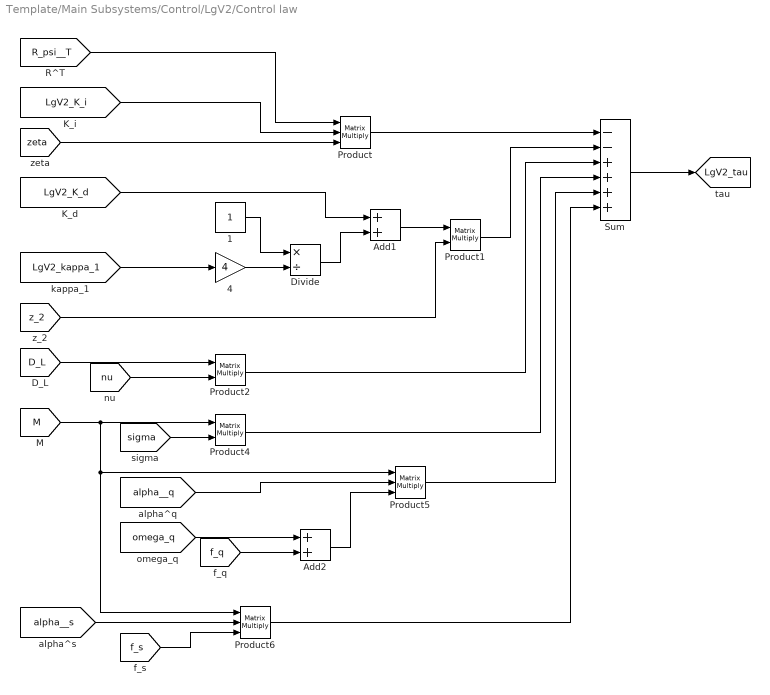
== system Template/Main Subsystems/Control/LgV2/Control law ==
  1 : Constant  OutDataType=fixdt(1, 16)  OutScaling=2^0
  4 : Gain  Gain=4  ParameterDataType=fixdt(1, 16)  ParameterScaling=2^0  OutDataType=fixdt(1, 16)  OutScaling=2^0
  Add1 : Sum  OutDataType=fixdt(1, 16)  OutScaling=2^-10
  Add2 : Sum  OutDataType=fixdt(1, 16)  OutScaling=2^-10
  Divide : Product  Inputs=*/  OutDataType=fixdt(1, 16)  OutScaling=2^-10
  Product : Product  Inputs=3  Multiplication=Matrix(*)  OutDataType=fixdt(1, 16)  OutScaling=2^0  RndMeth=Zero
  Product1 : Product  Multiplication=Matrix(*)  OutDataType=fixdt(1, 16)  OutScaling=2^0  RndMeth=Zero
  Product2 : Product  Multiplication=Matrix(*)  OutDataType=fixdt(1, 16)  OutScaling=2^0  RndMeth=Zero
  Product4 : Product  Multiplication=Matrix(*)  OutDataType=fixdt(1, 16)  OutScaling=2^0  RndMeth=Zero
  Product5 : Product  Inputs=3  Multiplication=Matrix(*)  OutDataType=fixdt(1, 16)  OutScaling=2^0  RndMeth=Zero
  Product6 : Product  Inputs=3  Multiplication=Matrix(*)  OutDataType=fixdt(1, 16)  OutScaling=2^0  RndMeth=Zero
  Sum : Sum  Inputs=--++++  OutDataType=fixdt(1, 16)  OutScaling=2^-10
  tag scope: LgV2_tau=global
  wires:
  Sum/1 -> [LgV2_tau]
  [R_psi__T] -> Product/1
  [LgV2_K_i] -> Product/2
  [zeta] -> Product/3
  [LgV2_K_d] -> Add1/1
  Divide/1 -> Add1/2
  1/1 -> Divide/1
  [LgV2_kappa_1] -> 4/1
  4/1 -> Divide/2
  Add1/1 -> Product1/1
  [z_2] -> Product1/2
  Product1/1 -> Sum/2
  [nu] -> Product2/2
  [D_L] -> Product2/1
  Product2/1 -> Sum/3
  [M] -> Product4/1, Product5/1, Product6/1
  [sigma] -> Product4/2
  Product4/1 -> Sum/4
  [alpha__q] -> Product5/2
  Product5/1 -> Sum/5
  [alpha__s] -> Product6/2
  [f_s] -> Product6/3
  Product6/1 -> Sum/6
  [omega_q] -> Add2/1
  [f_q] -> Add2/2
  Add2/1 -> Product5/3
  Product/1 -> Sum/1

== system Template/Main Subsystems/Control/LgV2/R(psi) ==
  psi : Inport
  -1 : Gain  Gain=-1  ParameterDataType=fixdt(1, 16)  ParameterScaling=2^0  OutDataType=fixdt(1, 16)  OutScaling=2^0
  Mux : Mux  Inputs=9
  R(psi) : Reshape  OutputDimensionality=Customize  OutputDimensions=[3,3]
  R11 : Trigonometry  Operator=cos
  R12 : Trigonometry
  R{13,23,31..32} (4 alike) : Constant  Value=0
  R21 : Trigonometry
  R22 : Trigonometry  Operator=cos
  R33 : Constant
  R : Outport
  tag scope: R_psi=global
  wires:
  R(psi)/1 -> R/1, [R_psi]
  Mux/1 -> R(psi)/1
  psi/1 -> R11/1, R21/1, R12/1, R22/1
  R11/1 -> Mux/1
  R21/1 -> Mux/2
  R31/1 -> Mux/3
  R12/1 -> -1/1
  R22/1 -> Mux/5
  R32/1 -> Mux/6
  R13/1 -> Mux/7
  R33/1 -> Mux/9
  R23/1 -> Mux/8
  -1/1 -> Mux/4

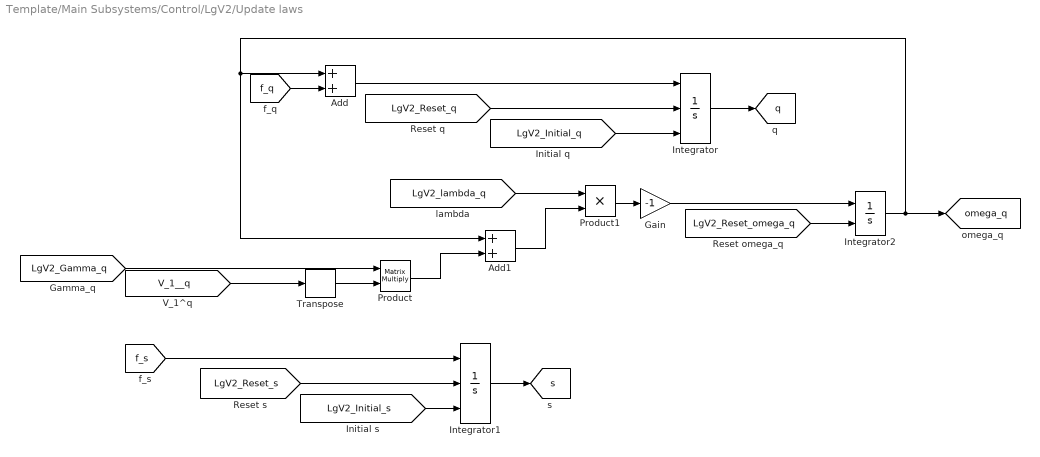
== system Template/Main Subsystems/Control/LgV2/Update laws ==
  Add : Sum  OutDataType=fixdt(1, 16)  OutScaling=2^-10
  Add1 : Sum  OutDataType=fixdt(1, 16)  OutScaling=2^-10
  Gain : Gain  Gain=-1  ParameterDataType=fixdt(1, 16)  ParameterScaling=2^0  OutDataType=fixdt(1, 16)  OutScaling=2^0
  Integrator : Integrator  ExternalReset=level  InitialConditionSource=external
  Integrator1 : Integrator  ExternalReset=level  InitialConditionSource=external  InitialCondition=250
  Integrator2 : Integrator  ExternalReset=level
  Product : Product  Multiplication=Matrix(*)  OutDataType=fixdt(1, 16)  OutScaling=2^0  RndMeth=Zero
  Product1 : Product  OutDataType=fixdt(1, 16)  OutScaling=2^0  RndMeth=Zero
  Transpose : dspmtrx3/Transpose  SystemSampleTime=-1  Hermitian=off  overflowFlag=off
  tag scope: omega_q=global, q=global, s=global
  wires:
  [f_q] -> Add/2
  Add/1 -> Integrator/1
  Product/1 -> Add1/2
  [V_1__q] -> Transpose/1
  [LgV2_Gamma_q] -> Product/1
  [LgV2_lambda_q] -> Product1/1
  Add1/1 -> Product1/2
  Product1/1 -> Gain/1
  Gain/1 -> Integrator2/1
  [f_s] -> Integrator1/1
  Transpose/1 -> Product/2
  Integrator/1 -> [q]
  Integrator1/1 -> [s]
  Integrator2/1 -> [omega_q], Add1/1, Add/1
  [LgV2_Reset_s] -> Integrator1/2
  [LgV2_Initial_s] -> Integrator1/3
  [LgV2_Reset_q] -> Integrator/2
  [LgV2_Initial_q] -> Integrator/3
  [LgV2_Reset_omega_q] -> Integrator2/2

== system Template/Main Subsystems/Control/LgV2/V_1^q ==
  Gain : Gain  Gain=-1  ParameterDataType=fixdt(1, 16)  ParameterScaling=2^0  OutDataType=fixdt(1, 16)  OutScaling=2^0
  Product : Product  Inputs=3  Multiplication=Matrix(*)  OutDataType=fixdt(1, 16)  OutScaling=2^0  RndMeth=Zero
  Transpose : dspmtrx3/Transpose  SystemSampleTime=-1  Hermitian=off  overflowFlag=off
  tag scope: V_1__q=global
  wires:
  Product/1 -> Gain/1
  [R_psi__T] -> Product/2
  [z_1] -> Transpose/1
  Transpose/1 -> Product/1
  [chi__q] -> Product/3
  Gain/1 -> [V_1__q]

== system Template/Main Subsystems/Control/LgV2/alpha ==
  Add : Sum  OutDataType=fixdt(1, 16)  OutScaling=2^-10
  I : dspmtrx3/Constant Diagonal Matrix  SystemSampleTime=-1  q=[1 1 1 ]  frame=off  dataType=Inherit from 'Constant(s) along diagonal'  isSigned=on  wordLen=16  udDataType=sfix(16)  fracBitsMode=Best precision  numFracBits=15
  Product : Product  OutDataType=fixdt(1, 16)  OutScaling=2^0  RndMeth=Zero
  Product1 : Product  Multiplication=Matrix(*)  OutDataType=fixdt(1, 16)  OutScaling=2^0  RndMeth=Zero
  Product2 : Product  Multiplication=Matrix(*)  OutDataType=fixdt(1, 16)  OutScaling=2^0  RndMeth=Zero
  Subtract : Sum  Inputs=+-  OutDataType=fixdt(1, 16)  OutScaling=2^-10
  Sum : Sum  Inputs=-+  OutDataType=fixdt(1, 16)  OutScaling=2^-10
  tag scope: alpha=global
  wires:
  Sum/1 -> [alpha]
  [LgV2_K_p] -> Subtract/1
  [LgV2_kappa_1] -> Product/1
  I/1 -> Product/2
  Product/1 -> Subtract/2
  Subtract/1 -> Product1/1
  [z_1] -> Product1/2
  Product1/1 -> Sum/1
  [R_psi__T] -> Product2/1
  [g_q] -> Add/1
  [g_s] -> Add/2
  Add/1 -> Product2/2
  Product2/1 -> Sum/2
